simulink model "Linearization2"  (R2022a)
settings: Solver=VariableStepAuto  StartTime=0.0  StopTime=10.0  RelTol=1e-3
undefined symbols (not defined in the file): Aactuator, ac, AeroCoeff, ControlAllocation, DUmax, DUmin, EngineTable, F, fcs, ft, g, hground, IC, kg, LandingGear, Light, LPmethod, m, MIL, Mode_deflection_aileron, Mode_deflection_elevator, Mode_deflection_rudder, Mode_deflection_TVC_y, Mode_deflection_TVC_z, N, Ninv_2nozzle, Ninv_no_nozzle, PIController, s, Sensor, slug, state0, sysID_DAQ, sysID_OBES, Umax_2nozzle, Umax_no_nozzle, Umin_2nozzle, Umin_no_nozzle, WMM2020
libraries: aerolibconvert2 x19, slpidlib x6, simulink x6, sharedutil x4, aerolibatmos2 x3, aerolibwind2 x3, aerolibbdyn x3, aerolibgravity2 x2, sharedtransform x1
(part 6 of 9)

== system Linearization2/F-16 Vehicle Systems Model/Vehicle/Propulsion/Thrust Vector Nozzle ZY1 ==
  note: ${\left[\begin{array}{c} F_x^{{\left(T\right)}} \\ F_y^{{\left(T\right)}} \\ F_z^{{\left(T\right)}} \end{array}\right]}={\left[\begin{array}{c} T_x \\ T_y \\ T_z \end{array}\right]}={\left[\begin{array}{c} T_{lx} \\ T_{ly} \\ T_{lz} \end{array}\right]}+{\left[\begin{array}{c} T_{rx} \\ T_{ry} \\ T_{rz} \end{array}\right]}=\frac{T}{2}{\left[\begin{array}{cc} & \cos \delta_{lz} \cos \delta_{ly} +\mathrm{cos}\delta_{rz} \cos \delta_{ry} \\ & \sin \delta_{lz} +\sin \delta_{rz} \\ - & \cos \delta_{lz} \sin \delta_{ly} -\cos \delta_{rz} \sin \delta_{ry} \end{array}\right]}$
  note: ${\left[\begin{array}{c} M_x^{{\left(T\right)}} \\ M_y^{{\left(T\right)}} \\ M_z^{{\left(T\right)}} \end{array}\right]}={\left[\begin{array}{c} M_{lx} \\ M_{ly} \\ M_{lz} \end{array}\right]}+{\left[\begin{array}{c} M_{rx} \\ M_{ry} \\ M_{rz} \end{array}\right]}=\frac{T}{2}{\left[\begin{array}{l} m_T \cos \delta_{lz} \sin \delta_{ly} -m_T \mathrm{cos}\delta_{rz} \sin \delta_{ry} \\ -l_T \cos \delta_{lz} \sin \delta_{ly} -l_T \mathrm{cos}\delta_{rz} \sin \delta_{ry} \\ {-l}_T \sin \delta_{lz} -l_T \sin \delta_{rz} \end{array}\right]}$
  note: 單一噴嘴的推力
  T1 : Inport
  Actuator (deg) : Inport  Port=2
  " lt1" : Inport  Port=3
  " mt" : Inport  Port=4
  Add{,1..2,4} (4 alike) : Sum
  Add3 : Sum  Inputs=+-
  Add5 : Sum  Inputs=--
  Angle Conversion{4..7} (4 alike) : aerolibconvert2/Angle Conversion  IU=deg  OU=rad
  Bus Selector1 : BusSelector  OutputSignals=TVC_rY_pitch_deg,TVC_rZ_yaw_deg,TVC_lY_pitch_deg,TVC_lZ_yaw_deg
  Constant1 : Constant  Value=-1
  Constant2 : Constant  Value=-1
  Cos{2..5} (4 alike) : Trigonometry  Operator=cos
  Mux2 : Mux  Inputs=6
  Product3 : Product  Inputs=3
  Product4 : Product  Inputs=3
  Product5 : Product
  Product6 : Product
  Product7 : Product  Inputs=4
  Product8 : Product  Inputs=4
  Sin{2..5} (4 alike) : Trigonometry
  pitch1 : Product
  pitch2 : Product
  roll1 : Product
  roll2 : Product
  yaw1 : Product
  yaw2 : Product
  FM : Outport  VectorParamsAs1DForOutWhenUnconnected=off
  Tx : Outport  Port=2  VectorParamsAs1DForOutWhenUnconnected=off
  Ty : Outport  Port=3  VectorParamsAs1DForOutWhenUnconnected=off
  Tz : Outport  Port=4  VectorParamsAs1DForOutWhenUnconnected=off
  wires:
  Add5/1 -> Mux2/6  "Mz"
  Cos2/1 -> Product3/2
  Product3/1 -> Add/1  "Trx"
  Cos3/1 -> Product7/2, Product3/3
  Angle Conversion5/1 -> Cos3/1, Sin3/1
  Angle Conversion4/1 -> Cos2/1, Sin2/1
  Actuator (deg)/1 -> Bus Selector1/1
  Bus Selector1/2 -> Angle Conversion5/1  "<TVC_rZ_yaw_deg>"
  T1/1 -> Product3/1, Product4/1, Product5/1, Product6/1, Product7/1, Product8/1  "T/2"
  Mux2/1 -> FM/1
  Bus Selector1/3 -> Angle Conversion6/1  "<TVC_lY_pitch_deg>"
  Bus Selector1/4 -> Angle Conversion7/1  "<TVC_lZ_yaw_deg>"
  Bus Selector1/1 -> Angle Conversion4/1  "<TVC_rY_pitch_deg>"
  Angle Conversion6/1 -> Cos4/1, Sin4/1
  Angle Conversion7/1 -> Sin5/1, Cos5/1
  Cos4/1 -> Product4/2
  Product4/1 -> Add/2  "Tlx"
  Cos5/1 -> Product8/2, Product4/3
  Add/1 -> Mux2/1, Tx/1  "axial thrust Tx"
  Sin3/1 -> Product5/2
  Sin5/1 -> Product6/2
  Product5/1 -> yaw1/1, Add1/1  "Try"
  Product6/1 -> Add1/2, yaw2/1  "Tly"
  Add1/1 -> Mux2/2, Ty/1  "yawing thrust Ty"
  Sin2/1 -> Product7/3
  Constant1/1 -> Product7/4
  Product7/1 -> roll1/1, pitch1/1, Add2/1  "Trz"
  Sin4/1 -> Product8/3
  Constant2/1 -> Product8/4
  Product8/1 -> pitch2/1, roll2/1, Add2/2  "Tlz"
  Add2/1 -> Tz/1, Mux2/3  "pitching thrust Tz"
  " mt"/1 -> roll2/2, roll1/2  "mt"
  roll1/1 -> Add3/1
  roll2/1 -> Add3/2
  Add3/1 -> Mux2/4  "Mx"
  " lt1"/1 -> yaw2/2, yaw1/2, pitch2/2, pitch1/2  "lt1"
  pitch1/1 -> Add4/1
  pitch2/1 -> Add4/2
  Add4/1 -> Mux2/5  "My"
  yaw1/1 -> Add5/1
  yaw2/1 -> Add5/2

== system Linearization2/F-16 Vehicle Systems Model/Vehicle/Propulsion(two_nozzles)/Actuators ==
  In Bus Element : Inport  PortName=Commands  Element=TVC_ry
  In Bus Element1 : Inport  PortName=Commands  Element=TVC_rz
  Gain4 : Gain  Gain=20.202  SaturateOnIntegerOverflow=on  OutDataTypeStr=Inherit: Same as input  ParamDataTypeStr=Inherit: Same as input
  Gain5 : Gain  Gain=20.202  SaturateOnIntegerOverflow=on  OutDataTypeStr=Inherit: Same as input  ParamDataTypeStr=Inherit: Same as input
  Rate Saturation4 : Saturate  UpperLimit=Aactuator.TVC_ry.RateLimitUpper  LowerLimit=Aactuator.TVC_ry.RateLimitLower
  Rate Saturation5 : Saturate  UpperLimit=Aactuator.TVC_rz.RateLimitUpper  LowerLimit=Aactuator.TVC_rz.RateLimitLower
  Sum4 : Sum  Inputs=|+-  InputSameDT=on  SaturateOnIntegerOverflow=on  OutDataTypeStr=Inherit: Same as first input
  Sum5 : Sum  Inputs=|+-  InputSameDT=on  SaturateOnIntegerOverflow=on  OutDataTypeStr=Inherit: Same as first input
  TVC_ry_AngleLimit : Saturate  UpperLimit=Aactuator.TVC_ry.AngleLimitUpper  LowerLimit=Aactuator.TVC_ry.AngleLimitLower
  TVC_ry_Integrator (degrees) : Integrator  InitialCondition=Aactuator.TVC_ry.IntegratorInitial  LimitOutput=on  UpperSaturationLimit=Aactuator.TVC_ry.AngleLimitUpper  LowerSaturationLimit=Aactuator.TVC_ry.AngleLimitLower
  TVC_rz_AngleLimit : Saturate  UpperLimit=Aactuator.TVC_rz.AngleLimitUpper  LowerLimit=Aactuator.TVC_rz.AngleLimitLower
  TVC_rz_Integrator (degrees) : Integrator  InitialCondition=Aactuator.TVC_rz.IntegratorInitial  LimitOutput=on  UpperSaturationLimit=Aactuator.TVC_rz.AngleLimitUpper  LowerSaturationLimit=Aactuator.TVC_rz.AngleLimitLower
  Out Bus Element : Outport  PortName=ActPositions  Element=TVC_ry_pitch_deg
  Out Bus Element1 : Outport  PortName=ActPositions  Element=TVC_rz_yaw_deg
  ActSensor_Out.TVC_ry_pitch_deg : Outport  Port=2
  ActSensor_Out.TVC_rz_yaw_deg : Outport  Port=3
  wires:
  Sum5/1 -> Gain5/1
  TVC_ry_Integrator (degrees)/1 -> Out Bus Element/1, ActSensor_Out.TVC_ry_pitch_deg/1, Sum4/2
  Sum4/1 -> Gain4/1
  In Bus Element1/1 -> TVC_rz_AngleLimit/1  "Commands_TVC_rz_yaw_deg"
  TVC_rz_Integrator (degrees)/1 -> ActSensor_Out.TVC_rz_yaw_deg/1, Out Bus Element1/1, Sum5/2
  In Bus Element/1 -> TVC_ry_AngleLimit/1  "Commands_TVC_ry_pitch_deg"
  Rate Saturation5/1 -> TVC_rz_Integrator (degrees)/1
  Gain4/1 -> Rate Saturation4/1
  Gain5/1 -> Rate Saturation5/1
  Rate Saturation4/1 -> TVC_ry_Integrator (degrees)/1
  TVC_ry_AngleLimit/1 -> Sum4/1
  TVC_rz_AngleLimit/1 -> Sum5/1

== system Linearization2/F-16 Vehicle Systems Model/Vehicle/Propulsion(two_nozzles)/Actuators1 ==
  In Bus Element4 : Inport  PortName=Commands  Element=TVC_ly
  In Bus Element2 : Inport  PortName=Commands  Element=TVC_lz
  Gain1 : Gain  Gain=20.202  SaturateOnIntegerOverflow=on  OutDataTypeStr=Inherit: Same as input  ParamDataTypeStr=Inherit: Same as input
  Gain2 : Gain  Gain=20.202  SaturateOnIntegerOverflow=on  OutDataTypeStr=Inherit: Same as input  ParamDataTypeStr=Inherit: Same as input
  Rate Saturation1 : Saturate  UpperLimit=Aactuator.TVC_ly.RateLimitUpper  LowerLimit=Aactuator.TVC_ly.RateLimitLower
  Rate Saturation2 : Saturate  UpperLimit=Aactuator.TVC_lz.RateLimitUpper  LowerLimit=Aactuator.TVC_lz.RateLimitLower
  Sum1 : Sum  Inputs=|+-  InputSameDT=on  SaturateOnIntegerOverflow=on  OutDataTypeStr=Inherit: Same as first input
  Sum2 : Sum  Inputs=|+-  InputSameDT=on  SaturateOnIntegerOverflow=on  OutDataTypeStr=Inherit: Same as first input
  TVC_ly_AngleLimit : Saturate  UpperLimit=Aactuator.TVC_ly.AngleLimitUpper  LowerLimit=Aactuator.TVC_ly.AngleLimitLower
  TVC_ly_Integrator (degrees) : Integrator  InitialCondition=Aactuator.TVC_ly.IntegratorInitial  LimitOutput=on  UpperSaturationLimit=Aactuator.TVC_ly.AngleLimitUpper  LowerSaturationLimit=Aactuator.TVC_ly.AngleLimitLower
  TVC_lz_AngleLimit : Saturate  UpperLimit=Aactuator.TVC_lz.AngleLimitUpper  LowerLimit=Aactuator.TVC_lz.AngleLimitLower
  TVC_lz_Integrator (degrees) : Integrator  InitialCondition=Aactuator.TVC_lz.IntegratorInitial  LimitOutput=on  UpperSaturationLimit=Aactuator.TVC_lz.AngleLimitUpper  LowerSaturationLimit=Aactuator.TVC_lz.AngleLimitLower
  Out Bus Element4 : Outport  PortName=ActPositions  Element=TVC_ly_pitch_deg
  Out Bus Element5 : Outport  PortName=ActPositions  Element=TVC_lz_yaw_deg
  ActSensor_Out.TVC_ly_pitch_deg : Outport  Port=2
  ActSensor_Out.TVC_lz_yaw_deg : Outport  Port=3
  wires:
  TVC_lz_Integrator (degrees)/1 -> ActSensor_Out.TVC_lz_yaw_deg/1, Out Bus Element5/1, Sum2/2
  Gain1/1 -> Rate Saturation1/1
  Gain2/1 -> Rate Saturation2/1
  Rate Saturation1/1 -> TVC_ly_Integrator (degrees)/1
  Rate Saturation2/1 -> TVC_lz_Integrator (degrees)/1
  Sum1/1 -> Gain1/1
  In Bus Element2/1 -> TVC_lz_AngleLimit/1  "Commands_TVC_lz_yaw_deg"
  Sum2/1 -> Gain2/1
  In Bus Element4/1 -> TVC_ly_AngleLimit/1  "Commands_TVC_ly_pitch_deg"
  TVC_ly_Integrator (degrees)/1 -> ActSensor_Out.TVC_ly_pitch_deg/1, Out Bus Element4/1, Sum1/2
  TVC_ly_AngleLimit/1 -> Sum1/1
  TVC_lz_AngleLimit/1 -> Sum2/1

== system Linearization2/F-16 Vehicle Systems Model/Vehicle/Propulsion(two_nozzles)/Afterburning Turbofan Jet Engine ==
  note: TODO: 發動機模型不完整，要看參考文獻進行更完整建模
  note: 參考文獻： Nguyen, T. Luat, et al., "Simulator Study of StallPost-Stall Characteristics of a Fighter Airplane with Relaxed Longitudinal Static Stability," NASA Technical Paper 1538 , Dec. 1979.
  note: $pow{\left(\delta_{th} \right)}={\left\{\begin{array}{c} 64.94\delta_{th} \ ,\\ 217.38\delta_{th} -117.38\ ,\ \ \ \end{array}\begin{array}{c} if{\mathrm{\ }\delta }_{th} \le 0.77\\ if{\mathrm{\ }\delta }_{th} >0.77 \end{array}\right)}$
  note: $T={\left\{\begin{array}{c} T_{idle} +{\left(T_{mil} -T_{idle} \right)}{\left(\frac{pow}{50}\right)},\ \ \ \ \ \ \ \ if\ pow<50\\ T_{mil} +{\left(T_{max} -T_{mil} \right)}{\left(\frac{pow-50}{50}\right)},\ \ \ if\ pow\ge 50 \end{array}\begin{array}{c} \ \\ \ \ \end{array}\right)}$
  note: 功率位準 power level
  note: 油門推桿位置 $0\le \delta_{th} \le 1$
  Mach : Inport
  H (ft) : Inport  Port=2
  Tc (lbf) : Inport  Port=3
  Add : Sum  Inputs=+-
  Add1 : Sum
  Add2 : Sum
  Constant : Constant
  Constant1 : Constant  Value=0
  Gain : Gain  Gain=64.94
  Gain1 : Gain  Gain=217.38
  If : If  IfExpression=u1<50  ElseIfExpressions=u1>=50  ShowElse=off
  If Action Subsystem : Subsystem  TreatAsAtomicUnit=on
  If Action Subsystem1 : Subsystem  TreatAsAtomicUnit=on
  If Action Subsystem2 : Subsystem  TreatAsAtomicUnit=on
  If Action Subsystem3 : Subsystem  TreatAsAtomicUnit=on
  If Action Subsystem4 : Subsystem  TreatAsAtomicUnit=on
  If Action Subsystem5 : Subsystem  TreatAsAtomicUnit=on
  If Action Subsystem6 : Subsystem  TreatAsAtomicUnit=on
  If1 : If  IfExpression=u1<50  ElseIfExpressions=u1>=50  ShowElse=off
  If2 : If  NumInputs=3  IfExpression=u3 == u1  ElseIfExpressions=u3>u1 & u3<=u2
  Merge : Merge  Inputs=3
  Mux : Mux  Inputs=2
  Mux1 : Mux  Inputs=2
  Mux4 : Mux  Inputs=5
  Saturation Dynamic : simulink/Discontinuities/Saturation Dynamic  OutMin=[]  OutMax=[]  OutDataTypeStr=Inherit: Same as second input  OutDataType=fixdt(1, 16)  OutScaling=2^-10  DoSatur=off
  Thrust Tidle : Interpolation_n-D  Table=EngineTable.idle  InternalRulePriority=Speed
  Thrust Tmax : Interpolation_n-D  Table=EngineTable.maximum  InternalRulePriority=Speed
  Thrust Tmil : Interpolation_n-D  Table=EngineTable.military  InternalRulePriority=Speed
  To Workspace : ToWorkspace  VariableName=T_max_min  SaveFormat=Timeseries  SampleTime=-1
  To Workspace1 : ToWorkspace  VariableName=check_engine  SaveFormat=Timeseries  SampleTime=-1
  To Workspace2 : ToWorkspace  VariableName=Mach_alt_input  SaveFormat=Timeseries  SampleTime=-1
  afterburner_off : Constant  Value=2
  afterburner_on : Constant  Value=3
  attitude Prelookup : PreLookup  BreakpointsData=EngineTable.attitude_Prelookup  IndexSearchMethod=Linear search  BeginIndexSearchUsingPreviousIndexResult=on  DiagnosticForOutOfRangeInput=Warning
  constant : Constant  Value=117.38
  idle : Constant
  mach Prelookup : PreLookup  BreakpointsData=EngineTable.mach_Prelookup  IndexSearchMethod=Linear search  BeginIndexSearchUsingPreviousIndexResult=on  DiagnosticForOutOfRangeInput=Warning
  T (lbf) : Outport  VectorParamsAs1DForOutWhenUnconnected=off
  engine_state : Outport  Port=2  VectorParamsAs1DForOutWhenUnconnected=off
  wires:
  Mach/1 -> mach Prelookup/1, Mux/2
  H (ft)/1 -> attitude Prelookup/1, Mux/1
  Add2/1 -> Saturation Dynamic/3, Mux1/2  "T_min"
  Add1/1 -> Saturation Dynamic/1, Mux1/1  "T_max"
  attitude Prelookup/2 -> Thrust Tmil/4, Thrust Tmax/4, Thrust Tidle/4
  Mux1/1 -> To Workspace/1
  Mux/1 -> To Workspace2/1
  Gain1/1 -> Add/1
  If Action Subsystem1/1(T_max1) -> Add1/2
  Constant/1 -> Gain1/1
  mach Prelookup/1 -> Thrust Tmil/1, Thrust Tmax/1, Thrust Tidle/1
  If/2 -> If Action Subsystem1/Action
  If1/2 -> If Action Subsystem3/Action
  If Action Subsystem3/1(T_min) -> Add2/2
  If Action Subsystem2/1(T_min) -> Add2/1
  If1/1 -> If Action Subsystem2/Action
  Gain/1 -> Mux4/2, If1/1  "pow"
  If Action Subsystem/1(T_max1) -> Add1/1
  mach Prelookup/2 -> Thrust Tmil/2, Thrust Tmax/2, Thrust Tidle/2
  Thrust Tidle/1 -> Mux4/3, If2/1  "Tidle"
  If/1 -> If Action Subsystem/Action
  Add/1 -> Mux4/1, If/1  "pow"
  constant/1 -> Add/2
  Mux4/1 -> If Action Subsystem1/1("input "), If Action Subsystem2/1("input "), If Action Subsystem3/1("input "), To Workspace1/1, If Action Subsystem/1("input ")
  Constant1/1 -> Gain/1
  attitude Prelookup/1 -> Thrust Tmil/3, Thrust Tmax/3, Thrust Tidle/3
  If2/1 -> If Action Subsystem4/Action
  If2/3 -> If Action Subsystem6/Action
  idle/1 -> If Action Subsystem4/1(In1)
  afterburner_on/1 -> If Action Subsystem6/1(In1)
  Thrust Tmil/1 -> If2/2, Mux4/4  "Tmil"
  Thrust Tmax/1 -> Mux4/5
  If Action Subsystem6/1(Out1) -> Merge/3
  If Action Subsystem5/1(Out1) -> Merge/2
  If Action Subsystem4/1(Out1) -> Merge/1
  afterburner_off/1 -> If Action Subsystem5/1(In1)
  If2/2 -> If Action Subsystem5/Action
  Saturation Dynamic/1 -> T (lbf)/1, If2/3  "Thrust (lbf)"
  Merge/1 -> engine_state/1
  Tc (lbf)/1 -> Saturation Dynamic/2

== system Linearization2/F-16 Vehicle Systems Model/Vehicle/Propulsion(two_nozzles)/Thrust Vector Nozzle ZY1 ==
  note: ${\left[\begin{array}{c} F_x^{{\left(T\right)}} \\ F_y^{{\left(T\right)}} \\ F_z^{{\left(T\right)}} \end{array}\right]}={\left[\begin{array}{c} T_x \\ T_y \\ T_z \end{array}\right]}={\left[\begin{array}{c} T_{lx} \\ T_{ly} \\ T_{lz} \end{array}\right]}+{\left[\begin{array}{c} T_{rx} \\ T_{ry} \\ T_{rz} \end{array}\right]}=\frac{T}{2}{\left[\begin{array}{cc} & \cos \delta_{lz} \cos \delta_{ly} +\mathrm{cos}\delta_{rz} \cos \delta_{ry} \\ & \sin \delta_{lz} +\sin \delta_{rz} \\ - & \cos \delta_{lz} \sin \delta_{ly} -\cos \delta_{rz} \sin \delta_{ry} \end{array}\right]}$
  note: ${\left[\begin{array}{c} M_x^{{\left(T\right)}} \\ M_y^{{\left(T\right)}} \\ M_z^{{\left(T\right)}} \end{array}\right]}={\left[\begin{array}{c} M_{lx} \\ M_{ly} \\ M_{lz} \end{array}\right]}+{\left[\begin{array}{c} M_{rx} \\ M_{ry} \\ M_{rz} \end{array}\right]}=\frac{T}{2}{\left[\begin{array}{l} m_T \cos \delta_{lz} \sin \delta_{ly} -m_T \mathrm{cos}\delta_{rz} \sin \delta_{ry} \\ -l_T \cos \delta_{lz} \sin \delta_{ly} -l_T \mathrm{cos}\delta_{rz} \sin \delta_{ry} \\ {-l}_T \sin \delta_{lz} -l_T \sin \delta_{rz} \end{array}\right]}$
  note: 單一噴嘴的推力
  T1 : Inport
  Actuator (deg) : Inport  Port=2
  " lt1" : Inport  Port=3
  " mt" : Inport  Port=4
  Angle Conversion4 : aerolibconvert2/Angle Conversion  IU=deg  OU=rad
  Angle Conversion5 : aerolibconvert2/Angle Conversion  IU=deg  OU=rad
  Bus Selector1 : BusSelector  OutputSignals=TVC_ry_pitch_deg,TVC_rz_yaw_deg
  Constant1 : Constant  Value=-1
  Constant2 : Constant  Value=-1
  Cos2 : Trigonometry  Operator=cos
  Cos3 : Trigonometry  Operator=cos
  Product3 : Product  Inputs=3
  Product5 : Product
  Product7 : Product  Inputs=4
  Sin2 : Trigonometry
  Sin3 : Trigonometry
  pitch1 : Product
  roll1 : Product
  yaw1 : Product  Inputs=3
  Trx : Outport  VectorParamsAs1DForOutWhenUnconnected=off
  Try : Outport  Port=2  VectorParamsAs1DForOutWhenUnconnected=off
  Trz : Outport  Port=3  VectorParamsAs1DForOutWhenUnconnected=off
  Mrx : Outport  Port=4  VectorParamsAs1DForOutWhenUnconnected=off
  Mry : Outport  Port=5  VectorParamsAs1DForOutWhenUnconnected=off
  Mrz : Outport  Port=6  VectorParamsAs1DForOutWhenUnconnected=off
  wires:
  yaw1/1 -> Mrz/1  "Mrz"
  Cos2/1 -> Product3/2
  Product3/1 -> Trx/1  "Trx"
  Cos3/1 -> Product7/2, Product3/3
  Angle Conversion5/1 -> Cos3/1, Sin3/1
  Angle Conversion4/1 -> Cos2/1, Sin2/1
  Actuator (deg)/1 -> Bus Selector1/1
  Bus Selector1/2 -> Angle Conversion5/1  "<TVC_rz_yaw_deg>"
  T1/1 -> Product3/1, Product5/1, Product7/1  "T/2"
  Bus Selector1/1 -> Angle Conversion4/1  "<TVC_ry_pitch_deg>"
  Sin3/1 -> Product5/2
  Product5/1 -> Try/1, yaw1/1  "Try"
  Sin2/1 -> Product7/3
  Constant1/1 -> Product7/4
  Product7/1 -> roll1/1, pitch1/1, Trz/1  "Trz"
  " mt"/1 -> roll1/2  "mt"
  roll1/1 -> Mrx/1  "Mrx"
  " lt1"/1 -> yaw1/2, pitch1/2  "lt1"
  pitch1/1 -> Mry/1  "Mry"
  Constant2/1 -> yaw1/3

== system Linearization2/F-16 Vehicle Systems Model/Vehicle/Propulsion(two_nozzles)/Thrust Vector Nozzle ZY2 ==
  note: ${\left[\begin{array}{c} F_x^{{\left(T\right)}} \\ F_y^{{\left(T\right)}} \\ F_z^{{\left(T\right)}} \end{array}\right]}={\left[\begin{array}{c} T_x \\ T_y \\ T_z \end{array}\right]}={\left[\begin{array}{c} T_{lx} \\ T_{ly} \\ T_{lz} \end{array}\right]}+{\left[\begin{array}{c} T_{rx} \\ T_{ry} \\ T_{rz} \end{array}\right]}=\frac{T}{2}{\left[\begin{array}{cc} & \cos \delta_{lz} \cos \delta_{ly} +\mathrm{cos}\delta_{rz} \cos \delta_{ry} \\ & \sin \delta_{lz} +\sin \delta_{rz} \\ - & \cos \delta_{lz} \sin \delta_{ly} -\cos \delta_{rz} \sin \delta_{ry} \end{array}\right]}$
  note: ${\left[\begin{array}{c} M_x^{{\left(T\right)}} \\ M_y^{{\left(T\right)}} \\ M_z^{{\left(T\right)}} \end{array}\right]}={\left[\begin{array}{c} M_{lx} \\ M_{ly} \\ M_{lz} \end{array}\right]}+{\left[\begin{array}{c} M_{rx} \\ M_{ry} \\ M_{rz} \end{array}\right]}=\frac{T}{2}{\left[\begin{array}{l} m_T \cos \delta_{lz} \sin \delta_{ly} -m_T \mathrm{cos}\delta_{rz} \sin \delta_{ry} \\ -l_T \cos \delta_{lz} \sin \delta_{ly} -l_T \mathrm{cos}\delta_{rz} \sin \delta_{ry} \\ {-l}_T \sin \delta_{lz} -l_T \sin \delta_{rz} \end{array}\right]}$
  note: 單一噴嘴的推力
  T1 : Inport
  Actuator (deg) : Inport  Port=2
  " lt1" : Inport  Port=3
  " mt" : Inport  Port=4
  Angle Conversion6 : aerolibconvert2/Angle Conversion  IU=deg  OU=rad
  Angle Conversion7 : aerolibconvert2/Angle Conversion  IU=deg  OU=rad
  Bus Selector1 : BusSelector  OutputSignals=TVC_ly_pitch_deg,TVC_lz_yaw_deg
  Constant1 : Constant  Value=-1
  Constant2 : Constant  Value=-1
  Constant3 : Constant  Value=-1
  Cos4 : Trigonometry  Operator=cos
  Cos5 : Trigonometry  Operator=cos
  Product4 : Product  Inputs=3
  Product6 : Product
  Product8 : Product  Inputs=4
  Sin4 : Trigonometry
  Sin5 : Trigonometry
  pitch2 : Product
  roll2 : Product  Inputs=3
  yaw2 : Product  Inputs=3
  Tlx : Outport  VectorParamsAs1DForOutWhenUnconnected=off
  Tly : Outport  Port=2  VectorParamsAs1DForOutWhenUnconnected=off
  Tlz : Outport  Port=3  VectorParamsAs1DForOutWhenUnconnected=off
  Mlx : Outport  Port=4  VectorParamsAs1DForOutWhenUnconnected=off
  Mly : Outport  Port=5  VectorParamsAs1DForOutWhenUnconnected=off
  Mlz : Outport  Port=6  VectorParamsAs1DForOutWhenUnconnected=off
  wires:
  yaw2/1 -> Mlz/1  "Mlz"
  Actuator (deg)/1 -> Bus Selector1/1
  T1/1 -> Product4/1, Product8/1, Product6/1  "T/2"
  Bus Selector1/1 -> Angle Conversion6/1  "<TVC_ly_pitch_deg>"
  Bus Selector1/2 -> Angle Conversion7/1  "<TVC_lz_yaw_deg>"
  Angle Conversion6/1 -> Cos4/1, Sin4/1
  Angle Conversion7/1 -> Sin5/1, Cos5/1
  Cos4/1 -> Product4/2
  Product4/1 -> Tlx/1  "Tlx"
  Cos5/1 -> Product8/2, Product4/3
  Sin5/1 -> Product6/2
  Product6/1 -> yaw2/1, Tly/1  "Tly"
  Sin4/1 -> Product8/3
  Constant2/1 -> Product8/4
  Product8/1 -> pitch2/1, roll2/1, Tlz/1  "Tlz"
  " mt"/1 -> roll2/2  "mt"
  roll2/1 -> Mlx/1  "Mlx"
  " lt1"/1 -> yaw2/2, pitch2/2  "lt1"
  pitch2/1 -> Mly/1  "Mly"
  Constant1/1 -> roll2/3
  Constant3/1 -> yaw2/3

== system Linearization2/F-16 Vehicle Systems Model/pqr NDI Controller/Control Allocation/CGIwrap ==
  IN_MAT : Inport
  Action Port : ActionPort  ActionPortLabel=elseif(u1 == 3)
  CGIwrap : MATLABFcn  MATLABFcn=CGIwrap
  Out1 : Outport
  wires:
  IN_MAT/1 -> CGIwrap/1
  CGIwrap/1 -> Out1/1

== system Linearization2/F-16 Vehicle Systems Model/pqr NDI Controller/Control Allocation/CGIwrap1 ==
  IN_MAT : Inport
  Action Port : ActionPort  ActionPortLabel=else
  CGIwrap : MATLABFcn  MATLABFcn=CGIwrap
  Out1 : Outport
  wires:
  IN_MAT/1 -> CGIwrap/1
  CGIwrap/1 -> Out1/1

== system Linearization2/F-16 Vehicle Systems Model/pqr NDI Controller/Control Allocation/DAISY_CHAINING ==
  IN_MAT : Inport
  Action Port : ActionPort  ActionPortLabel=elseif(u1 == 2)
  DAISY_CHAINING : MATLABFcn  MATLABFcn=DAISY_CHAINING
  Out1 : Outport
  wires:
  IN_MAT/1 -> DAISY_CHAINING/1
  DAISY_CHAINING/1 -> Out1/1

== system Linearization2/F-16 Vehicle Systems Model/pqr NDI Controller/Control Allocation/DA_Allocation ==
  IN_MAT : Inport
  Action Port : ActionPort  ActionPortLabel=elseif(u1 == 4)
  DA_Allocation : MATLABFcn  MATLABFcn=DA_Allocation
  Out1 : Outport
  wires:
  IN_MAT/1 -> DA_Allocation/1
  DA_Allocation/1 -> Out1/1

== system Linearization2/F-16 Vehicle Systems Model/pqr NDI Controller/Control Allocation/LPwrap_def1 ==
  IN_MAT : Inport
  Action Port : ActionPort  ActionPortLabel=elseif(u1==6)
  LPwrap_def1 : MATLABFcn  MATLABFcn=LPwrap_def1
  Out1 : Outport
  wires:
  IN_MAT/1 -> LPwrap_def1/1
  LPwrap_def1/1 -> Out1/1

== system Linearization2/F-16 Vehicle Systems Model/pqr NDI Controller/Control Allocation/LPwrap_lift ==
  IN_MAT : Inport
  Action Port : ActionPort  ActionPortLabel=elseif(u1==7)
  LPwrap_lift : MATLABFcn  MATLABFcn=LPwrap_lift
  Out1 : Outport
  wires:
  IN_MAT/1 -> LPwrap_lift/1
  LPwrap_lift/1 -> Out1/1

== system Linearization2/F-16 Vehicle Systems Model/pqr NDI Controller/Control Allocation/LPwrap_sig ==
  IN_MAT : Inport
  Action Port : ActionPort  ActionPortLabel=elseif(u1==8)
  LPwrap_sig : MATLABFcn  MATLABFcn=LPwrap_sig
  Out1 : Outport
  wires:
  IN_MAT/1 -> LPwrap_sig/1
  LPwrap_sig/1 -> Out1/1

== system Linearization2/F-16 Vehicle Systems Model/pqr NDI Controller/Control Allocation/LPwrap_thrust ==
  IN_MAT : Inport
  Action Port : ActionPort  ActionPortLabel=elseif(u1==9)
  LPwrap_thrust : MATLABFcn  MATLABFcn=LPwrap_thrust
  Out1 : Outport
  wires:
  IN_MAT/1 -> LPwrap_thrust/1
  LPwrap_thrust/1 -> Out1/1

== system Linearization2/F-16 Vehicle Systems Model/pqr NDI Controller/Control Allocation/Pseudo_inverses_ShunYuanChang2019 ==
  note: 控制配置： 聯動式
  y_bar : Inport
  g1 : Inport  Port=2
  N : Inport  Port=3
  Action Port : ActionPort  ActionPortLabel=elseif(u1==10)
  Control Allocation : MATLAB Function  TreatAsAtomicUnit=on
  Output : Outport
  wires:
  y_bar/1 -> Control Allocation/1(y_bar)
  g1/1 -> Control Allocation/2(g1)
  N/1 -> Control Allocation/3(N)
  Control Allocation/1(u_bar) -> Output/1

== system Linearization2/F-16 Vehicle Systems Model/pqr NDI Controller/Control Allocation/Weighted_Pseudo_inverses ==
  IN_MAT : Inport
  Action Port : ActionPort  ActionPortLabel=if(u1 == 1)
  Weighted_Pseudo_inverses : MATLABFcn  MATLABFcn=Weighted_Pseudo_inverses
  Out1 : Outport
  wires:
  IN_MAT/1 -> Weighted_Pseudo_inverses/1
  Weighted_Pseudo_inverses/1 -> Out1/1

== system Linearization2/F-16 Vehicle Systems Model/pqr NDI Controller/Control Allocation/control_management ==
  IN_MAT : Inport
  Action Port : ActionPort  ActionPortLabel=elseif(u1 == 5)
  control_management : MATLABFcn  MATLABFcn=control_management
  Out1 : Outport
  wires:
  IN_MAT/1 -> control_management/1
  control_management/1 -> Out1/1

== system Linearization2/F-16 Vehicle Systems Model/pqr NDI Controller/control matrix g1/Pitching  ==
  note: $g_{q_{\delta_{re} } } =g_{q_{\delta_{le} } } =\frac{\begin{array}{l} \overset{-}{q} S\overset{-}{C} {\left\{{\left(\frac{{\hat{m} }_{\delta_e } }{2}+{\left(x_{cg,ref} -x_{cg} \right)}∙\frac{{\hat{Z} }_{\delta_e } }{2}\right\}}\right)} \end{array}\mathrm}{I_y }$
  note: 註：因為 $\delta$ 單位是度(degree)，所以需要額外用 ${\left(\frac{\pi }{180°}\right)}$ 做單位換算
  note: $g_{q_{\delta_{ry} } } =\frac{-l_T }{I_y }\frac{T}{2}∙{\left(\frac{\pi }{180°}\right)}$
  note: 有指定port dimensions=[1,9]
  note: 1  gp_dra1
      |     gp_dla1
      |     gp_dre1
      |     gp_dle1
      |     gp_dr1
      |     gp_dra2
      |     gp_dla2
      |     gp_dre2
      |     gp_dle2
      |     gp_dr2
      |
      | 11 gq_dra
      |      gq_dla
      |      gq_dre
      |      gq_dle
      |
      | 15 gr_dra1
      |      gr_dla1
      |      gr_dre1
      |      gr_dle1
      |      gr_dr1
      |      gr_dra2
      |      gr_dla2
      |      gr_dre2
      |      gr_dle2
      |      gr_dr2
  note: 33 lt1
  note: 32 T/2
  note: 34 mt
  note: ${\hat{m} }_{\delta_e } =\frac{1}{0.2}{\left[\ C_m {\left(\alpha ,\beta ,\delta_e +0.1°\right)}{∙\eta }_{\delta_e } {\left(\delta_e +0.1°\right)}+\Delta C_{m_{ds} } {\left(\alpha ,\delta_e +0.1°\right)}\right)}+{\left(x_{cg,ref} -x_{cg} \right)}∙C_Z {\left(\alpha ,\beta ,\delta_e +0.1°\right)}$
  note: $-C_m {\left(\alpha ,\beta ,\delta_e -0.1°\right)}{∙\eta }_{\delta_e } {\left(\delta_e -0.1°\right)}-\Delta C_{m_{ds} } {\left(\alpha ,\delta_e -0.1°\right)}-{\left(x_{cg,ref} -x_{cg} \right)}∙C_Z {\left(\alpha ,\beta ,\delta_e -0.1°\right)}\rbrack}$
  note: 25 m
      | 26 Ix
      | 27 Iy
      | 28 Iz
      | 29 Ixy
      | 30 Ixz
      | 31 Iyz
  note: $g_1 {\left({\overset{-}{x} }_1 \right)}={\left[\begin{array}{ccccccccc} g_{p_{\delta_{ra} } } & g_{p_{\delta_{la} } } & g_{p_{\delta_{re} } } & g_{p_{\delta_{le} } } & g_{p_{\delta_r } } & g_{p_{\delta_{ry} } } & g_{p_{\delta_{rz} } } & g_{p_{\delta_{ly} } } & g_{p_{\delta_{lz} } } \\ g_{q_{\delta_{ra} } } & g_{q_{\delta_{la} } } & g_{q_{\delta_{re} } } & g_{q_{\delta_{le} } } & 0 & g_{q_{\delta_{ry} } } & 0 & g_{q_{\delta_{ly} } } & 0 \\ g_{r_{\delta_{ra} } } & g_{r_{\delta_{la} } } & g_{r_{\delta_{re} } } & g_{r_{\delta_{le} } } & g_{r_{\delta_r } } & g_{r_{\delta_{ry} } } & g_{r_{\delta_{rz} } } & g_{r_{\delta_{ly} } } & g_{r_{\delta_{lz} } } \end{array}\right]}$
  note: $g_{q_{\delta_{ly} } } =\frac{-l_T }{I_y }\frac{T}{2}∙{\left(\frac{\pi }{180°}\right)}$
  control_g : Inport
  inertia : Inport  Port=2
  Thrust : Inport  Port=3
  lt1 : Inport  Port=4
  mt : Inport  Port=5
  Mux : Mux  Inputs=5
  Mux1 : Mux  Inputs=9
  g(2,5) : Constant  Value=0
  pitch with TVC_lY : Fcn  Expr=( -1*u(33)*u(32) ) / u(27) *pi/180
  pitch with TVC_lZ : Constant  Value=0
  pitch with TVC_rY : Fcn  Expr=( -1*u(33)*u(32) ) / u(27) *pi/180
  pitch with TVC_rZ : Constant  Value=0
  "pitch with left Elevator " : Fcn  Expr=u(14)/u(27)
  pitch with left aileron : Fcn  Expr=u(12)/u(27)
  "pitch with right Elevator " : Fcn  Expr=u(13)/u(27)
  pitch with right aileron : Fcn  Expr=u(11)/u(27)
  g1 Row2 : Outport  PortDimensions=[1,9]  VectorParamsAs1DForOutWhenUnconnected=off
  wires:
  control_g/1 -> Mux/1
  Mux1/1 -> g1 Row2/1
  inertia/1 -> Mux/2
  Thrust/1 -> Mux/3
  lt1/1 -> Mux/4
  Mux/1 -> "pitch with right Elevator "/1, pitch with right aileron/1, pitch with left aileron/1, "pitch with left Elevator "/1, pitch with TVC_lY/1, pitch with TVC_rY/1
  g(2,5)/1 -> Mux1/5
  pitch with TVC_rY/1 -> Mux1/6
  pitch with TVC_rZ/1 -> Mux1/7
  "pitch with left Elevator "/1 -> Mux1/4
  "pitch with right Elevator "/1 -> Mux1/3
  pitch with left aileron/1 -> Mux1/2
  pitch with right aileron/1 -> Mux1/1
  pitch with TVC_lY/1 -> Mux1/8
  pitch with TVC_lZ/1 -> Mux1/9
  mt/1 -> Mux/5

== system Linearization2/F-16 Vehicle Systems Model/pqr NDI Controller/control matrix g1/Rolling  ==
  note: $g_{p_{\delta_{ra} } } =\frac{1}{I_x I_z {-I}_{xz}^2 }{\left\{I_z \;∙\;g_{p_{\delta_{ra1} } }+I_{xz} \;∙\;g_{p_{\delta_{ra2} } }\right\}}$
  note: 註：因為 $\delta$ 單位是度(degree)，所以需要額外用 ${\left(\frac{\pi }{180°}\right)}$ 做單位換算
  note: $g_{p_{\delta_{rz} } } =\frac{-I_{xz} l_T }{I_x I_z -I_{xz}^2 }\frac{T}{2}∙{\left(\frac{\pi }{180°}\right)}$
  note: 33 lt1
  note: 25 m
      | 26 Ix
      | 27 Iy
      | 28 Iz
      | 29 Ixy
      | 30 Ixz
      | 31 Iyz
  note: 32 T/2
  note: 有指定port dimensions=[1,9]
  note: 34 mt
  note: $g_{p_{\delta_{la} } } =\frac{1}{I_x I_z {-I}_{xz}^2 }{\left\{I_z \;∙\;g_{p_{\delta_{la1} } }+I_{xz} \;∙\;g_{p_{\delta_{la2} } }\right\}}$
  note: $g_{p_{\delta_{re} } } =\frac{1}{I_x I_z {-I}_{xz}^2 }{\left\{I_z \;∙\;g_{p_{\delta_{re1} } }+I_{xz} \;∙\;g_{p_{\delta_{re2} } }\right\}}$
  note: $g_{p_{\delta_{le} } } =\frac{1}{I_x I_z {-I}_{xz}^2 }{\left\{I_z \;∙\;g_{p_{\delta_{le1} } }+I_{xz} \;∙\;g_{p_{\delta_{le2} } }\right\}}$
  note: $g_{p_{\delta_{r} } } =\frac{1}{I_x I_z {-I}_{xz}^2 }{\left\{I_z \;∙\;g_{p_{\delta_{r1} } }+I_{xz} \;∙\;g_{p_{\delta_{r2} } }\right\}}$
  note: $g_{r_{\delta_{re2} } } =g_{p_{\delta_{re2} } }$
  note: $g_{r_{\delta_{la2} } } =g_{p_{\delta_{la2} } }$
  note: $=\begin{array}{l} \overset{-}{q} Sb{\left\{{\left(C_{n_{\delta_{re} } } -{\left(x_{cg,ref} -x_{cg} \right)}∙\frac{\overset{-}{C} }{b}∙\Delta C_{Y_{\delta_e } } \right\}}\right)} \end{array}∙{\left(\frac{1}{25°}\right)}$
  note: $g_{r_{\delta_{ra2} } } =g_{p_{\delta_{ra2} } }$
  note: $=-\begin{array}{l} \overset{-}{q} Sb{\left\{{\left(\frac{{\left[\Delta C_{n_{\delta_a } } +\Delta C_{n_{{\delta_a }_{LEF} } } ∙{\left(1-\frac{\delta_{LEF} }{25°}\right)}\right]}}{2}-\frac{{\left[\Delta C_{Y_{\delta_a } } +\Delta C_{Y_{{\delta_a }_{LEF} } } ∙{\left(1-\frac{\delta_{LEF} }{25°}\right)}\right]}}{2}∙{\left(x_{cg,ref} -x_{cg} \right)}∙\frac{\overset{-}{C} }{b}\right\}}\right)} \end{array}∙{\left(\frac{1}{20°}\right)}$
  note: $g_{r_{\delta_{le2} } } =g_{p_{\delta_{le2} } }$
  note: $=\begin{array}{l} \overset{-}{q} Sb{\left\{{\left(\frac{{\left[\Delta C_{n_{\delta_a } } +\Delta C_{n_{{\delta_a }_{LEF} } } ∙{\left(1-\frac{\delta_{LEF} }{25°}\right)}\right]}}{2}-\frac{{\left[\Delta C_{Y_{\delta_a } } +\Delta C_{Y_{{\delta_a }_{LEF} } } ∙{\left(1-\frac{\delta_{LEF} }{25°}\right)}\right]}}{2}∙{\left(x_{cg,ref} -x_{cg} \right)}∙\frac{\overset{-}{C} }{b}\right\}}\right)} \end{array}∙{\left(\frac{1}{20°}\right)}$
  note: $=\begin{array}{l} -\overset{-}{q} Sb{\left\{{\left(C_{n_{\delta_{le} } } -{\left(x_{cg,ref} -x_{cg} \right)}∙\frac{\overset{-}{C} }{b}∙\Delta C_{Y_{\delta_e } } \right\}}\right)} \end{array}∙{\left(\frac{1}{25°}\right)}$
  note: $g_{r_{\delta_{r 2}} } =g_{p_{\delta_{r2} }$
  note: $=\bar{q} Sb∙\Delta C_{l_{\delta_r } } ∙{\left(\frac{1}{30°}\right)}$
  note: $=\begin{array}{l} \overset{-}{q} Sb{\left\{{\left(C_{l_{\delta_{re} } } \right\}}\right)} \end{array}∙{\left(\frac{1}{25°}\right)}$
  note: $=\bar{q} Sb∙{\left[\Delta C_{n_{\delta_r } } -{\left(x_{cg,ref} -x_{cg} \right)}∙\frac{\bar{c} }{b}∙\Delta C_{Y_{\delta_r } } \right]}∙{\left(\frac{1}{30°}\right)}$
  note: $g_{r_{\delta_r 1} } =g_{p_{\delta_r 1} }$
  note: $=\begin{array}{l} -\overset{-}{q} Sb{\left\{{\left(C_{l_{\delta_{le} } } \right\}}\right)} \end{array}∙{\left(\frac{1}{25°}\right)}$
  note: $g_{r_{\delta_{re1} } } =g_{p_{\delta_{re1} } }$
  note: $=\begin{array}{l} \overset{-}{q} Sb{\left\{{\left(\frac{{\left[\Delta C_{l_{\delta_a } } +\Delta C_{l_{{\delta_a }_{LEF} } } ∙{\left(1-\frac{\delta_{LEF} }{25°}\right)}\right]}}{2}\right\}}\right)} \end{array}∙{\left(\frac{1}{20°}\right)}$
  note: $g_{r_{\delta_{la1} } } =g_{p_{\delta_{la1} } }$
  note: $g_{r_{\delta_{ra1} } } =g_{p_{\delta_{ra1} } }$
  note: $=-\begin{array}{l} \overset{-}{q} Sb{\left\{{\left(\frac{{\left[\Delta C_{l_{\delta_a } } +\Delta C_{l_{{\delta_a }_{LEF} } } ∙{\left(1-\frac{\delta_{LEF} }{25°}\right)}\right]}}{2}\right\}}\right)} \end{array}∙{\left(\frac{1}{20°}\right)}$
  note: $g_{r_{\delta_{le1} } }=g_{p_{\delta_{le1} } }$
  note: 1  gp_dra1
      | 2  gp_dla1
      | 3  gp_dre1
      | 4  gp_dle1
      | 5  gp_dr1
      | 6  gp_dra2
      | 7  gp_dla2
      | 8  gp_dre2
      | 9  gp_dle2
      | 10 gp_dr2
      |
      | 11 gq_dra
      | 12 gq_dla
      | 13 gq_dre
      | 14 gq_dle
      |
      | 15 gr_dra1
      | 16  gr_dla1
      | 17  gr_dre1
      | 18  gr_dle1
      | 19  gr_dr1
      | 20  gr_dra2
      | 21  gr_dla2
      | 22  gr_dre2
      | 23  gr_dle2
      | 24  gr_dr2
  note: $g_{p_{\delta_{ry} } } =\frac{-I_z m_T }{I_x I_z -I_{xz}^2 }\frac{T}{2}∙{\left(\frac{\pi }{180°}\right)}$
  note: $g_{p_{\delta_{ly} } } =\frac{I_z m_T }{I_x I_z -I_{xz}^2 }\frac{T}{2}∙{\left(\frac{\pi }{180°}\right)}$
  note: $g_{p_{\delta_{lz} } } =\frac{-I_{xz} l_T }{I_x I_z -I_{xz}^2 }\frac{T}{2}∙{\left(\frac{\pi }{180°}\right)}$
  note: $g_1 {\left({\overset{-}{x} }_1 \right)}={\left[\begin{array}{ccccccccc} g_{p_{\delta_{ra} } } & g_{p_{\delta_{la} } } & g_{p_{\delta_{re} } } & g_{p_{\delta_{le} } } & g_{p_{\delta_r } } & g_{p_{\delta_{ry} } } & g_{p_{\delta_{rz} } } & g_{p_{\delta_{ly} } } & g_{p_{\delta_{lz} } } \\ g_{q_{\delta_{ra} } } & g_{q_{\delta_{la} } } & g_{q_{\delta_{re} } } & g_{q_{\delta_{le} } } & 0 & g_{q_{\delta_{ry} } } & 0 & g_{q_{\delta_{ly} } } & 0 \\ g_{r_{\delta_{ra} } } & g_{r_{\delta_{la} } } & g_{r_{\delta_{re} } } & g_{r_{\delta_{le} } } & g_{r_{\delta_r } } & g_{r_{\delta_{ry} } } & g_{r_{\delta_{rz} } } & g_{r_{\delta_{ly} } } & g_{r_{\delta_{lz} } } \end{array}\right]}$
  control_g : Inport
  inertia : Inport  Port=2
  Thrust : Inport  Port=3
  lt1 : Inport  Port=4
  mt : Inport  Port=5
  Mux : Mux  Inputs=5
  Mux1 : Mux  Inputs=9
  roll with TVC_lY : Fcn  Expr="(  u(28)*u(32)*u(34)  ) /  ( u(26)*u(28)-u(30)^2  ) *pi/180"
  roll with TVC_lZ : Fcn  Expr="(  -1*u(30)*u(32)*u(33)  ) /  ( u(26)*u(28)-u(30)^2  ) *pi/180"
  roll with TVC_rY : Fcn  Expr="( -1* u(28)*u(32)*u(34)  ) /  ( u(26)*u(28)-u(30)^2  ) *pi/180"
  roll with TVC_rZ : Fcn  Expr="(  -1*u(30)*u(32)*u(33)  ) /  ( u(26)*u(28)-u(30)^2  ) *pi/180"
  roll with left aileron : Fcn  Expr=( ( u(28)*u(2)+u(30)*u(7) ) / ( u(26)*u(28)-u(30)^2 ) )
  roll with left elevator : Fcn  Expr=( ( u(28)*u(4)+u(30)*u(9) ) / ( u(26)*u(28)-u(30)^2 ) )
  roll with right aileron : Fcn  Expr=( ( u(28)*u(1)+u(30)*u(6) ) / ( u(26)*u(28)-u(30)^2 ) )
  roll with right elevator : Fcn  Expr=( ( u(28)*u(3)+u(30)*u(8) ) / ( u(26)*u(28)-u(30)^2 ) )
  "roll with rudder " : Fcn  Expr=( ( u(28)*u(5)+u(30)*u(10) ) / ( u(26)*u(28)-u(30)^2 ) )
  g1 Row1 : Outport  PortDimensions=[1,9]  VectorParamsAs1DForOutWhenUnconnected=off
  wires:
  control_g/1 -> Mux/1
  Mux/1 -> roll with left aileron/1, roll with right aileron/1, roll with right elevator/1, roll with TVC_rY/1, roll with TVC_rZ/1, roll with TVC_lZ/1, roll with TVC_lY/1, "roll with rudder "/1, roll with left elevator/1
  Mux1/1 -> g1 Row1/1
  inertia/1 -> Mux/2
  Thrust/1 -> Mux/3
  lt1/1 -> Mux/4
  roll with right aileron/1 -> Mux1/1
  roll with left aileron/1 -> Mux1/2
  roll with right elevator/1 -> Mux1/3
  roll with left elevator/1 -> Mux1/4
  "roll with rudder "/1 -> Mux1/5
  roll with TVC_rY/1 -> Mux1/6
  mt/1 -> Mux/5
  roll with TVC_rZ/1 -> Mux1/7
  roll with TVC_lY/1 -> Mux1/8
  roll with TVC_lZ/1 -> Mux1/9

== system Linearization2/F-16 Vehicle Systems Model/pqr NDI Controller/control matrix g1/Yawing  ==
  note: 註：因為 $\delta$ 單位是度(degree)，所以需要額外用 ${\left(\frac{\pi }{180°}\right)}$ 做單位換算
  note: $g_{r_{\delta_{rz} } } =\frac{-I_x l_T }{I_x I_z -I_{xz}^2 }\frac{T}{2}∙{\left(\frac{\pi }{180°}\right)}$
  note: 有指定port dimensions=[1,9]
  note: 1  gp_dra1
      | 2  gp_dla1
      | 3  gp_dre1
      | 4  gp_dle1
      | 5  gp_dr1
      | 6  gp_dra2
      | 7  gp_dla2
      | 8  gp_dre2
      | 9  gp_dle2
      | 10 gp_dr2
      |
      | 11 gq_dra
      | 12 gq_dla
      | 13 gq_dre
      | 14 gq_dle
      |
      | 15 gr_dra1
      | 16  gr_dla1
      | 17  gr_dre1
      | 18  gr_dle1
      | 19  gr_dr1
      | 20  gr_dra2
      | 21  gr_dla2
      | 22  gr_dre2
      | 23  gr_dle2
      | 24  gr_dr2
  note: 32 T/2
  note: 33 lt1
  note: 34 mt
  note: $g_{p_{\delta_r } } =\frac{1}{I_x I_z {-I}_{xz}^2 }{\left(I_{xz} \;∙\;g_{r_{\delta_{r1} } }+I_{x} \;∙\;g_{r_{\delta_{r2} } }\right)}$
  note: $g_{r_{\delta_{ra} } } =\frac{1}{I_x I_z {-I}_{xz}^2 }{\left\{I_{xz} \;∙\;g_{r_{\delta_{ra1} } }+I_{x} \;∙\;g_{r_{\delta_{ra2} } }\right\}}$
  note: $g_{r_{\delta_{re} } } =\frac{1}{I_x I_z {-I}_{xz}^2 }{\left\{I_{xz} \;∙\;g_{r_{\delta_{re1} } }+I_{x} \;∙\;g_{r_{\delta_{re2} } }\right\}}$
  note: $g_{r_{\delta_{le} } } =\frac{1}{I_x I_z {-I}_{xz}^2 }{\left\{I_{xz} \;∙\;g_{r_{\delta_{le1} } }+I_{x} \;∙\;g_{r_{\delta_{le2} } }\right\}}$
  note: $g_{r_{\delta_{la} } } =\frac{1}{I_x I_z {-I}_{xz}^2 }{\left\{I_{xz} \;∙\;g_{r_{\delta_{la1} } }+I_{x} \;∙\;g_{r_{\delta_{la2} } }\right\}}$
  note: $=-\begin{array}{l} \overset{-}{q} Sb{\left\{{\left(\frac{{\left[\Delta C_{n_{\delta_a } } +\Delta C_{n_{{\delta_a }_{LEF} } } ∙{\left(1-\frac{\delta_{LEF} }{25°}\right)}\right]}}{2}-\frac{{\left[\Delta C_{Y_{\delta_a } } +\Delta C_{Y_{{\delta_a }_{LEF} } } ∙{\left(1-\frac{\delta_{LEF} }{25°}\right)}\right]}}{2}∙{\left(x_{cg,ref} -x_{cg} \right)}∙\frac{\overset{-}{C} }{b}\right\}}\right)} \end{array}∙{\left(\frac{1}{20°}\right)}$
  note: $g_{r_{\delta_{r 2}} } =g_{p_{\delta_{r2} }$
  note: $=\begin{array}{l} -\overset{-}{q} Sb{\left\{{\left(C_{n_{\delta_{le} } } -{\left(x_{cg,ref} -x_{cg} \right)}∙\frac{\overset{-}{C} }{b}∙\Delta C_{Y_{\delta_e } } \right\}}\right)} \end{array}∙{\left(\frac{1}{25°}\right)}$
  note: $=\begin{array}{l} \overset{-}{q} Sb{\left\{{\left(\frac{{\left[\Delta C_{n_{\delta_a } } +\Delta C_{n_{{\delta_a }_{LEF} } } ∙{\left(1-\frac{\delta_{LEF} }{25°}\right)}\right]}}{2}-\frac{{\left[\Delta C_{Y_{\delta_a } } +\Delta C_{Y_{{\delta_a }_{LEF} } } ∙{\left(1-\frac{\delta_{LEF} }{25°}\right)}\right]}}{2}∙{\left(x_{cg,ref} -x_{cg} \right)}∙\frac{\overset{-}{C} }{b}\right\}}\right)} \end{array}∙{\left(\frac{1}{20°}\right)}$
  note: $=\bar{q} Sb∙{\left[\Delta C_{n_{\delta_r } } -{\left(x_{cg,ref} -x_{cg} \right)}∙\frac{\bar{c} }{b}∙\Delta C_{Y_{\delta_r } } \right]}∙{\left(\frac{1}{30°}\right)}$
  note: $g_{r_{\delta_{le2} } } =g_{p_{\delta_{le2} } }$
  note: $g_{r_{\delta_{ra2} } } =g_{p_{\delta_{ra2} } }$
  note: $g_{r_{\delta_{re2} } } =g_{p_{\delta_{re2} } }$
  note: $g_{r_{\delta_{la2} } } =g_{p_{\delta_{la2} } }$
  note: $=\begin{array}{l} \overset{-}{q} Sb{\left\{{\left(C_{n_{\delta_{re} } } -{\left(x_{cg,ref} -x_{cg} \right)}∙\frac{\overset{-}{C} }{b}∙\Delta C_{Y_{\delta_e } } \right\}}\right)} \end{array}∙{\left(\frac{1}{25°}\right)}$
  note: $g_{r_{\delta_{la1} } } =g_{p_{\delta_{la1} } }$
  note: $g_{r_{\delta_{le1} } }=g_{p_{\delta_{le1} } }$
  note: $g_{r_{\delta_{ra1} } } =g_{p_{\delta_{ra1} } }$
  note: $g_{r_{\delta_{re1} } } =g_{p_{\delta_{re1} } }$
  note: $=\begin{array}{l} -\overset{-}{q} Sb{\left\{{\left(C_{l_{\delta_{le} } } \right\}}\right)} \end{array}∙{\left(\frac{1}{25°}\right)}$
  note: $g_{r_{\delta_r 1} } =g_{p_{\delta_r 1} }$
  note: $=-\begin{array}{l} \overset{-}{q} Sb{\left\{{\left(\frac{{\left[\Delta C_{l_{\delta_a } } +\Delta C_{l_{{\delta_a }_{LEF} } } ∙{\left(1-\frac{\delta_{LEF} }{25°}\right)}\right]}}{2}\right\}}\right)} \end{array}∙{\left(\frac{1}{20°}\right)}$
  note: $=\bar{q} Sb∙\Delta C_{l_{\delta_r } } ∙{\left(\frac{1}{30°}\right)}$
  note: $=\begin{array}{l} \overset{-}{q} Sb{\left\{{\left(C_{l_{\delta_{re} } } \right\}}\right)} \end{array}∙{\left(\frac{1}{25°}\right)}$
  note: $=\begin{array}{l} \overset{-}{q} Sb{\left\{{\left(\frac{{\left[\Delta C_{l_{\delta_a } } +\Delta C_{l_{{\delta_a }_{LEF} } } ∙{\left(1-\frac{\delta_{LEF} }{25°}\right)}\right]}}{2}\right\}}\right)} \end{array}∙{\left(\frac{1}{20°}\right)}$
  note: 25 m
      | 26 Ix
      | 27 Iy
      | 28 Iz
      | 29 Ixy
      | 30 Ixz
      | 31 Iyz
  note: $g_{r_{\delta_{ry} } } =\frac{-I_{xz} m_T }{I_x I_z -I_{xz}^2 }\frac{T}{2}∙{\left(\frac{\pi }{180°}\right)}$
  note: $g_{r_{\delta_{lz} } } =\frac{-I_x l_T }{I_x I_z -I_{xz}^2 }\frac{T}{2}∙{\left(\frac{\pi }{180°}\right)}$
  note: $g_{r_{\delta_{ly} } } =\frac{I_{xz} m_T }{I_x I_z -I_{xz}^2 }\frac{T}{2}∙{\left(\frac{\pi }{180°}\right)}$
  note: $g_1 {\left({\overset{-}{x} }_1 \right)}={\left[\begin{array}{ccccccccc} g_{p_{\delta_{ra} } } & g_{p_{\delta_{la} } } & g_{p_{\delta_{re} } } & g_{p_{\delta_{le} } } & g_{p_{\delta_r } } & g_{p_{\delta_{ry} } } & g_{p_{\delta_{rz} } } & g_{p_{\delta_{ly} } } & g_{p_{\delta_{lz} } } \\ g_{q_{\delta_{ra} } } & g_{q_{\delta_{la} } } & g_{q_{\delta_{re} } } & g_{q_{\delta_{le} } } & 0 & g_{q_{\delta_{ry} } } & 0 & g_{q_{\delta_{ly} } } & 0 \\ g_{r_{\delta_{ra} } } & g_{r_{\delta_{la} } } & g_{r_{\delta_{re} } } & g_{r_{\delta_{le} } } & g_{r_{\delta_r } } & g_{r_{\delta_{ry} } } & g_{r_{\delta_{rz} } } & g_{r_{\delta_{ly} } } & g_{r_{\delta_{lz} } } \end{array}\right]}$
  control_g : Inport
  inertia : Inport  Port=2
  Thrust : Inport  Port=3
  "lt1 " : Inport  Port=4
  mt : Inport  Port=5
  Mux : Mux  Inputs=5
  Mux1 : Mux  Inputs=9
  yaw with TVC_lY : Fcn  Expr="(  u(30)*u(32)*u(34)  ) / ( u(26)*u(28)-u(30)^2 ) *pi/180"
  yaw with TVC_lZ : Fcn  Expr="(  -1*u(26)*u(32)*u(33)  ) / ( u(26)*u(28)-u(30)^2 ) *pi/180"
  yaw with TVC_rY : Fcn  Expr="(  -1*u(30)*u(32)*u(34)  ) / ( u(26)*u(28)-u(30)^2 ) *pi/180"
  yaw with TVC_rZ : Fcn  Expr="(  -1*u(26)*u(32)*u(33)  ) / ( u(26)*u(28)-u(30)^2 ) *pi/180"
  yaw with left aileron : Fcn  Expr=( ( u(30)*u(16)+u(26)*u(21) ) / ( u(26)*u(28)-u(30)^2 ) )
  yaw with left elevator : Fcn  Expr=( ( u(30)*u(18)+u(26)*u(23) ) / ( u(26)*u(28)-u(30)^2 ) )
  yaw with right aileron : Fcn  Expr=( ( u(30)*u(15)+u(26)*u(20) ) / ( u(26)*u(28)-u(30)^2 ) )
  yaw with right elevator : Fcn  Expr=( ( u(30)*u(17)+u(26)*u(22) ) / ( u(26)*u(28)-u(30)^2 ) )
  yaw with rudder : Fcn  Expr=( ( u(30)*u(19)+u(26)*u(24) ) / ( u(26)*u(28)-u(30)^2 ) )
  g1 Row3 : Outport  PortDimensions=[1,9]  VectorParamsAs1DForOutWhenUnconnected=off
  wires:
  control_g/1 -> Mux/1
  Mux1/1 -> g1 Row3/1
  inertia/1 -> Mux/2
  Thrust/1 -> Mux/3
  yaw with right aileron/1 -> Mux1/1
  "lt1 "/1 -> Mux/4
  Mux/1 -> yaw with TVC_rY/1, yaw with TVC_rZ/1, yaw with TVC_lZ/1, yaw with TVC_lY/1, yaw with rudder/1, yaw with left aileron/1, yaw with right aileron/1, yaw with right elevator/1, yaw with left elevator/1
  yaw with left aileron/1 -> Mux1/2
  yaw with right elevator/1 -> Mux1/3
  yaw with left elevator/1 -> Mux1/4
  yaw with rudder/1 -> Mux1/5
  yaw with TVC_rY/1 -> Mux1/6
  yaw with TVC_rZ/1 -> Mux1/7
  yaw with TVC_lY/1 -> Mux1/8
  yaw with TVC_lZ/1 -> Mux1/9
  mt/1 -> Mux/5

== system Linearization2/F-16 Vehicle Systems Model/sysID_Onboard_Excitation_System/signal generator/Pause Counter ==
  note: "Output when disabled" 設成 reset
      | 且 "Initial output" 設成 1
      | 目的是為了當 Enable = 0 時，令計數器重設為輸出 1
  note: "States when enabling" 設成 reset
      | 目的是為了當 Enable = 0 時，能將計數器重設成為1
  note: Pause Counter
  note: 內部有設定：
      | 1. sysID_OBES.Ts
      | 2. 計數器的初始值
  note: 計數器的累加值
  note: 具有暫停計數功能的計數器
  note: 允許計數的最大值
  note: 計數到最大值時，就暫停計數(+0)；
      | 否則，就繼續計數
  note: 參考資料： https://www.youtube.com/watch?v=utj-NZ5Hb6U
      | How to Design a Counter (Up/Down/Reset/Pause) in Simulink/MATLAB
  Enable : EnablePort  StatesWhenEnabling=reset
  Add : Sum
  Constant : Constant  Value=sysID_OBES.TVC_ry.size
  Constant2 : Constant  Value=0
  Constant3 : Constant
  Relational Operator : RelationalOperator  Operator===  OutDataTypeStr=boolean  RndMeth=Simplest  InputSameDT=off
  Switch : Switch  Criteria=u2 ~= 0  SaturateOnIntegerOverflow=off  InputSameDT=off
  Unit Delay : UnitDelay  SampleTime=sysID_OBES.Ts  HasFrameUpgradeWarning=on
  CountValue : Outport  OutputWhenDisabled=reset  InitialOutput=1
  isCountDone : Outport  Port=2
  wires:
  Add/1 -> CountValue/1, Unit Delay/1
  Relational Operator/1 -> isCountDone/1, Switch/2
  Constant/1 -> Relational Operator/1
  Unit Delay/1 -> Add/2, Relational Operator/2
  Switch/1 -> Add/1
  Constant2/1 -> Switch/1
  Constant3/1 -> Switch/3

== system Linearization2/F-16 Vehicle Systems Model/sysID_Onboard_Excitation_System/signal generator1/Pause Counter ==
  note: "Output when disabled" 設成 reset
      | 且 "Initial output" 設成 1
      | 目的是為了當 Enable = 0 時，令計數器重設為輸出 1
  note: "States when enabling" 設成 reset
      | 目的是為了當 Enable = 0 時，能將計數器重設成為1
  note: Pause Counter
  note: 內部有設定：
      | 1. sysID_OBES.Ts
      | 2. 計數器的初始值
  note: 計數器的累加值
  note: 具有暫停計數功能的計數器
  note: 允許計數的最大值
  note: 計數到最大值時，就暫停計數(+0)；
      | 否則，就繼續計數
  note: 參考資料： https://www.youtube.com/watch?v=utj-NZ5Hb6U
      | How to Design a Counter (Up/Down/Reset/Pause) in Simulink/MATLAB
  Enable : EnablePort  StatesWhenEnabling=reset
  Add : Sum
  Constant : Constant  Value=sysID_OBES.TVC_rz.size
  Constant2 : Constant  Value=0
  Constant3 : Constant
  Relational Operator : RelationalOperator  Operator===  OutDataTypeStr=boolean  RndMeth=Simplest  InputSameDT=off
  Switch : Switch  Criteria=u2 ~= 0  SaturateOnIntegerOverflow=off  InputSameDT=off
  Unit Delay : UnitDelay  SampleTime=sysID_OBES.Ts  HasFrameUpgradeWarning=on
  CountValue : Outport  OutputWhenDisabled=reset  InitialOutput=1
  isCountDone : Outport  Port=2
  wires:
  Add/1 -> CountValue/1, Unit Delay/1
  Relational Operator/1 -> isCountDone/1, Switch/2
  Constant/1 -> Relational Operator/1
  Unit Delay/1 -> Add/2, Relational Operator/2
  Switch/1 -> Add/1
  Constant2/1 -> Switch/1
  Constant3/1 -> Switch/3

== system Linearization2/F-16 Vehicle Systems Model/sysID_Onboard_Excitation_System/signal generator2/Pause Counter ==
  note: "Output when disabled" 設成 reset
      | 且 "Initial output" 設成 1
      | 目的是為了當 Enable = 0 時，令計數器重設為輸出 1
  note: "States when enabling" 設成 reset
      | 目的是為了當 Enable = 0 時，能將計數器重設成為1
  note: Pause Counter
  note: 內部有設定：
      | 1. sysID_OBES.Ts
      | 2. 計數器的初始值
  note: 計數器的累加值
  note: 具有暫停計數功能的計數器
  note: 允許計數的最大值
  note: 計數到最大值時，就暫停計數(+0)；
      | 否則，就繼續計數
  note: 參考資料： https://www.youtube.com/watch?v=utj-NZ5Hb6U
      | How to Design a Counter (Up/Down/Reset/Pause) in Simulink/MATLAB
  Enable : EnablePort  StatesWhenEnabling=reset
  Add : Sum
  Constant : Constant  Value=sysID_OBES.TVC_ly.size
  Constant2 : Constant  Value=0
  Constant3 : Constant
  Relational Operator : RelationalOperator  Operator===  OutDataTypeStr=boolean  RndMeth=Simplest  InputSameDT=off
  Switch : Switch  Criteria=u2 ~= 0  SaturateOnIntegerOverflow=off  InputSameDT=off
  Unit Delay : UnitDelay  SampleTime=sysID_OBES.Ts  HasFrameUpgradeWarning=on
  CountValue : Outport  OutputWhenDisabled=reset  InitialOutput=1
  isCountDone : Outport  Port=2
  wires:
  Add/1 -> CountValue/1, Unit Delay/1
  Relational Operator/1 -> isCountDone/1, Switch/2
  Constant/1 -> Relational Operator/1
  Unit Delay/1 -> Add/2, Relational Operator/2
  Switch/1 -> Add/1
  Constant2/1 -> Switch/1
  Constant3/1 -> Switch/3

== system Linearization2/F-16 Vehicle Systems Model/sysID_Onboard_Excitation_System/signal generator3/Pause Counter ==
  note: "Output when disabled" 設成 reset
      | 且 "Initial output" 設成 1
      | 目的是為了當 Enable = 0 時，令計數器重設為輸出 1
  note: "States when enabling" 設成 reset
      | 目的是為了當 Enable = 0 時，能將計數器重設成為1
  note: Pause Counter
  note: 內部有設定：
      | 1. sysID_OBES.Ts
      | 2. 計數器的初始值
  note: 計數器的累加值
  note: 具有暫停計數功能的計數器
  note: 允許計數的最大值
  note: 計數到最大值時，就暫停計數(+0)；
      | 否則，就繼續計數
  note: 參考資料： https://www.youtube.com/watch?v=utj-NZ5Hb6U
      | How to Design a Counter (Up/Down/Reset/Pause) in Simulink/MATLAB
  Enable : EnablePort  StatesWhenEnabling=reset
  Add : Sum
  Constant : Constant  Value=sysID_OBES.TVC_lz.size
  Constant2 : Constant  Value=0
  Constant3 : Constant
  Relational Operator : RelationalOperator  Operator===  OutDataTypeStr=boolean  RndMeth=Simplest  InputSameDT=off
  Switch : Switch  Criteria=u2 ~= 0  SaturateOnIntegerOverflow=off  InputSameDT=off
  Unit Delay : UnitDelay  SampleTime=sysID_OBES.Ts  HasFrameUpgradeWarning=on
  CountValue : Outport  OutputWhenDisabled=reset  InitialOutput=1
  isCountDone : Outport  Port=2
  wires:
  Add/1 -> CountValue/1, Unit Delay/1
  Relational Operator/1 -> isCountDone/1, Switch/2
  Constant/1 -> Relational Operator/1
  Unit Delay/1 -> Add/2, Relational Operator/2
  Switch/1 -> Add/1
  Constant2/1 -> Switch/1
  Constant3/1 -> Switch/3

== system Linearization2/F-16 Vehicle Systems Model/sysID_Onboard_Excitation_System/signal generator4/Pause Counter ==
  note: "Output when disabled" 設成 reset
      | 且 "Initial output" 設成 1
      | 目的是為了當 Enable = 0 時，令計數器重設為輸出 1
  note: "States when enabling" 設成 reset
      | 目的是為了當 Enable = 0 時，能將計數器重設成為1
  note: Pause Counter
  note: 內部有設定：
      | 1. sysID_OBES.Ts
      | 2. 計數器的初始值
  note: 計數器的累加值
  note: 具有暫停計數功能的計數器
  note: 允許計數的最大值
  note: 計數到最大值時，就暫停計數(+0)；
      | 否則，就繼續計數
  note: 參考資料： https://www.youtube.com/watch?v=utj-NZ5Hb6U
      | How to Design a Counter (Up/Down/Reset/Pause) in Simulink/MATLAB
  Enable : EnablePort  StatesWhenEnabling=reset
  Add : Sum
  Constant : Constant  Value=sysID_OBES.right_aileron.size
  Constant2 : Constant  Value=0
  Constant3 : Constant
  Relational Operator : RelationalOperator  Operator===  OutDataTypeStr=boolean  RndMeth=Simplest  InputSameDT=off
  Switch : Switch  Criteria=u2 ~= 0  SaturateOnIntegerOverflow=off  InputSameDT=off
  Unit Delay : UnitDelay  SampleTime=sysID_OBES.Ts  HasFrameUpgradeWarning=on
  CountValue : Outport  OutputWhenDisabled=reset  InitialOutput=1
  isCountDone : Outport  Port=2
  wires:
  Add/1 -> CountValue/1, Unit Delay/1
  Relational Operator/1 -> isCountDone/1, Switch/2
  Constant/1 -> Relational Operator/1
  Unit Delay/1 -> Add/2, Relational Operator/2
  Switch/1 -> Add/1
  Constant2/1 -> Switch/1
  Constant3/1 -> Switch/3
